simulink model "DisturbSimulation"  (R2019a)
settings: Solver=ode45  StartTime=0.0  StopTime=100.0*60  RelTol=1e-8  AbsTol=1e-8
values from neighbouring files (symbols this model uses):
  Areas = [ APanelx , APanelx , APanelx , APanelx , APanely , APanely , APanelz, APanelz , APanelz , APanelz , ASensorx , ASensorx , ASensory , ASensory, ASensorz , ABusx , ABusx , ABusy , ABusy , ABuszp ,ABuszn ]    [SetUp.m]
  eps0 = quat0(2:4)    [SetUp.m]
  eta0 = quat0(1)    [SetUp.m]
  I = [ Ix 0 0 ; 0 Iy 0 ; 0 0 Iz ]    [SetUp.m]
  Norms = [nx     nx      -nx     -nx     ny      -ny     nz      nz      -nz     -nz     nx      -nx     ny      -ny     nz      nx      -nx     ny      -ny     nz      -nz     ]    [SetUp.m]
  Positions = [PPxp1 PPxp2 PPxn1 PPxn2 PPyp PPyn PPzp1 PPzp2 PPzn1 PPzn2 PSxp PSxn PSyp PSyn PSzp PBxp PBxn PByp PByn PBzp PBzn ] - COM    [SetUp.m]
  UTC = [ 2019 , 3 , 19 , 12 , 0 , 0 ]    [SetUp.m]
undefined symbols (not defined in the file or in its folder): r0, v0
libraries: sharedtransform x1
settings Model: Creator=liamh  LastModifiedBy=liamh

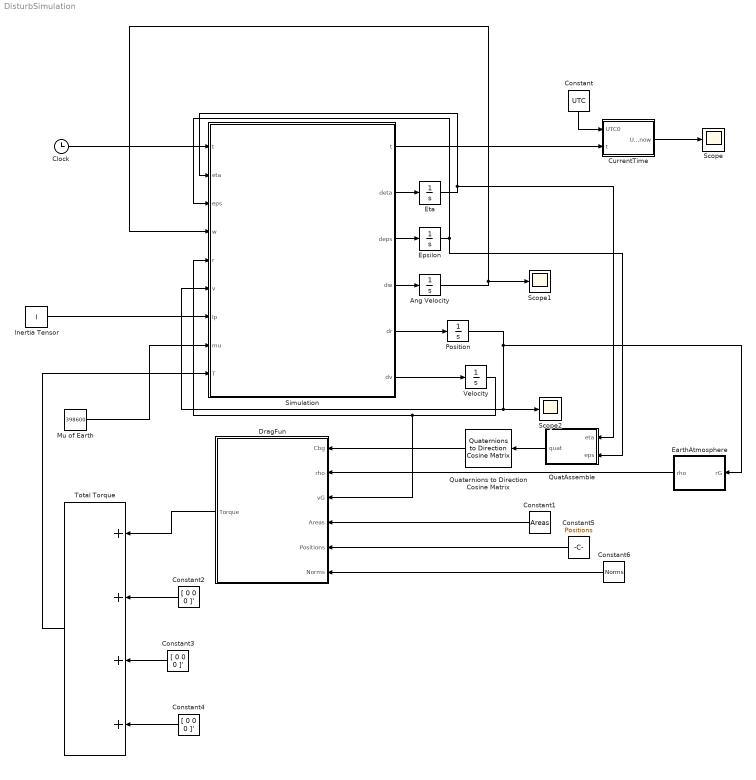
== system DisturbSimulation ==
  Ang Velocity : Integrator  InitialCondition=[ 0 -0.001047 0 ]'
  Clock : Clock
  Constant : Constant  Value=UTC  VectorParams1D=off
  Constant1 : Constant  Value=Areas
  Constant2 : Constant  Value=[ 0 0 0 ]'
  Constant3 : Constant  Value=[ 0 0 0 ]'
  Constant4 : Constant  Value=[ 0 0 0 ]'
  Constant5 : Constant  Value=Positions
  Constant6 : Constant  Value=Norms
  CurrentTime : MATLAB Function  TreatAsAtomicUnit=on
  DragFun : MATLAB Function  TreatAsAtomicUnit=on
  EarthAtmosphere : MATLAB Function  TreatAsAtomicUnit=on
  Epsilon : Integrator  InitialCondition=eps0
  "Eta " : Integrator  InitialCondition=eta0  ContinuousStateAttributes='eta'
  Inertia Tensor : Constant  Value=I  VectorParams1D=off
  "Mu of Earth " : Constant  Value=398600
  Position : Integrator  InitialCondition=r0
  QuatAssemble : MATLAB Function  TreatAsAtomicUnit=on
  Quaternions to Direction Cosine Matrix : sharedtransform/Quaternions to  Direction Cosine Matrix  aMode=aMode
      settings: SourceProductName=Aerospace Blockset  SourceProductBaseCode=AE
  Scope : Scope
  Scope1 : Scope
  Scope2 : Scope
  Simulation : MATLAB Function  TreatAsAtomicUnit=on
  Total Torque : Sum  Inputs=++++
  Velocity : Integrator  InitialCondition=v0
  wires:
  Inertia Tensor/1 -> Simulation/7(Ip)
  Simulation/2(deta) -> "Eta "/1
  Simulation/3(deps) -> Epsilon/1
  Simulation/4(dw) -> Ang Velocity/1
  Simulation/5(dr) -> Position/1
  Simulation/6(dv) -> Velocity/1
  "Mu of Earth "/1 -> Simulation/8(mu)
  Clock/1 -> Simulation/1("t ")
  Simulation/1(t) -> CurrentTime/2(t)
  Total Torque/1 -> Simulation/9(T)
  Constant/1 -> CurrentTime/1(UTC0)
  CurrentTime/1(UTCnow) -> Scope/1
  Ang Velocity/1 -> Scope1/1, Simulation/4(w)
  Constant4/1 -> Total Torque/4
  Constant3/1 -> Total Torque/3
  Constant2/1 -> Total Torque/2
  DragFun/1(Torque) -> Total Torque/1
  "Eta "/1 -> QuatAssemble/1(eta), Simulation/2(eta)
  Epsilon/1 -> Simulation/3(eps), QuatAssemble/2(eps)
  Velocity/1 -> Simulation/6(v)
  Position/1 -> EarthAtmosphere/1(rG), Scope2/1, DragFun/3(vG), Simulation/5(r)
  Constant6/1 -> DragFun/6(Norms)
  Constant5/1 -> DragFun/5(Positions)
  Constant1/1 -> DragFun/4(Areas)
  Quaternions to Direction Cosine Matrix/1 -> DragFun/1(Cbg)
  QuatAssemble/1(quat) -> Quaternions to Direction Cosine Matrix/1
  EarthAtmosphere/1(rho) -> DragFun/2(rho)

== matlab function DisturbSimulation/DragFun ==
  data: Cbg input; rho input; Torque output; vG input; Areas input; Positions input; Norms input
function Torque  = DragFun( Cbg , rho , vG , Areas , Positions , Norms )
% Velocity and Position are pulled in as an ECI value
vnorm = norm(vG)*1000 ; % m/s Magnitude of velocity
% The normal vectors on the body frame are pulled in
% Use rotation matrix to rotate from ECI to Bodyframe
vb = Cbg*vG ; %rotates the velocity vector into the body frame
% Model of Atmosphere
% Find the amount of area on each side, exposed to the sun, use dot products
Top = [0;0;0] ; %Preallocates Cps Parts 
Bot = 0 ; 
Drag = 0*vb ;
    for pp = 1:length(Areas)
        dotted = (Norms(:,pp)'*vb) ; %Dot product of norm and sun
        if dotted > 0 
            Drag = Drag + -rho*vnorm^2*vb*dotted*Areas(pp) ;
        end 
        % Need Center of Pressure Now
        if dotted > 0 
            Top = Top + Positions(:,pp) * dotted * Areas(pp) ; % Sums the position vector times the dotted value and area
            Bot = Bot + dotted * Areas(pp) ; %Sums the n dot s * area
        end
    end
Cps = Top/Bot ; %Defines the center of pressure
Torque = cross(Cps,Drag) ; %Cross product of force and distance

end

== matlab function DisturbSimulation/Simulation ==
  data: t output; t input; deta output; eta input; eps input; w input; r input; v input; Ip input; mu input; deps output; dw output; dr output; dv output; T input
function [ t , deta , deps , dw , dr , dv ]   = Simulation( t , eta , eps , w , r , v , Ip , mu , T )
% ( t , eta , eps , w , r , v , Ip , Avec , Day0 , mbar , UTC , mu)
% Simulates an attitude of s/c in LEO. State is quaternion [ eta , eps ]
% followed by angular velocity
    
% Find change in quaternions
    deps = .5 * ( eta*eye(3)*w + cross(eps,w) ) ;
    deta = -.5 * eps' * w ;
    
% Find change in angular velocity from torques 
    wcross = [ 0 -w(3) w(2) ; w(3) 0 -w(1) ; -w(2) w(1) 0 ] ;
    dw = T - wcross*Ip*w ;
    
% New ECI state vectors
    rad = norm( r ) ; %radius
    dr = v ;
    dv = -mu*r/rad^3 ;

== matlab function DisturbSimulation/CurrentTime ==
  data: UTC0 input; UTCnow output; t input
function UTCnow = CurrentTime( UTC0 , t )
     if t >= 60
         tmin = floor( t/60 ) ;
         t = t - tmin*60 ;
         if tmin >= 60
             thour = floor( tmin/60 ) ;
             tmin = tmin - thour*60 ;
         else
             thour = 0 ;
         end
     else
         tmin = 0 ;
         thour = 0 ;
     end
     if ( thour + UTC0(4) ) >= 24 
         thour = thour - 24 ;
         UTC0(3) = UTC0(3) + 1 ;
     end
     UTCnow = UTC0 + [ 0 0 0 thour tmin t ] ;

== matlab function DisturbSimulation/QuatAssemble ==
  data: eta input; quat output; eps input
function quat = QuatAssemble(eta,eps)
quat = [ eta , eps' ]' ;

== matlab function DisturbSimulation/EarthAtmosphere ==
  data: rG input; rho output
    function rho  = EarthStdAtm(rG)
    alt = (norm(rG) - 6378) ; %km - altitude of spacecraft
    
    % Chart Values Provided by the website below
    % http://toughsf.blogspot.com/2017/09/low-earth-orbit-atmospheric-scoops.html
    Altitudes = [50 60 70 80 100 200 300 400 500 600 700 800 900 1000] ; % Chart altitudes in km
    Densities = [1.03E-3 3.10E-4 8.28E-5 1.85E-5 5.36E-7 3.13E-10 2.40E-11 3.38E-12 6.21E-13 1.39E-13 4.03E-14 1.66E-14 9.11E-15 5.85E-15] ; %Densities for given altitudes in kg/m^3
    % Use linear interpolation
    Pos = find(Altitudes>alt) ;
    if alt>1000
        rho = 0 ;
    end
    Dens1 = Densities(Pos(1)) ; %Finds the density that is right below input
    Dens2 = Densities(Pos(1)+1) ; %Finds density above input altitude
    AltDiff = Altitudes(Pos(1)+1)-Altitudes(Pos(1)) ; % Finds Difference in altitudes
    rho = Dens1 + (Dens2-Dens1)/AltDiff ; %Linearly interpolates the rho at a given altitude

    end
